simulink model "ISC_laboratorio_02_ex3"  (R2019a)
settings: Solver=VariableStepAuto  StartTime=0.0  StopTime=20  RelTol=1e-3
settings Model: Creator=guilh  LastModifiedBy=guilh

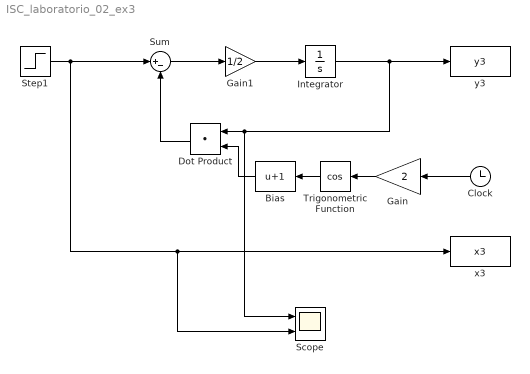
== system ISC_laboratorio_02_ex3 ==
  Bias : Bias  Bias=1
  Clock : Clock
  Dot Product : DotProduct  InputSameDT=on  OutDataTypeStr=Inherit: Inherit via internal rule
  Gain : Gain  Gain=2
  Gain1 : Gain  Gain=1/2
  Integrator : Integrator  InitialCondition=1
  Scope : Scope  NumInputPorts=2
  Step1 : Step  Time=0  SampleTime=0
  Sum : Sum  Inputs=|+-
  Trigonometric Function : Trigonometry  Operator=cos
  x3 : ToWorkspace  VariableName=x3  SampleTime=-1
  "y3 " : ToWorkspace  VariableName=y3  SampleTime=-1
  wires:
  Integrator/1 -> Scope/1, Dot Product/1, "y3 "/1
  Sum/1 -> Gain1/1
  Step1/1 -> Sum/1, Scope/2, x3/1
  Gain1/1 -> Integrator/1
  Gain/1 -> Trigonometric Function/1
  Clock/1 -> Gain/1
  Trigonometric Function/1 -> Bias/1
  Bias/1 -> Dot Product/2
  Dot Product/1 -> Sum/2
